simulink library "AF_MDL"  (R2015a)
settings: Solver=ode45  StartTime=0.0  StopTime=10.0  RelTol=1e-3
undefined symbols (not defined in the file or in its folder): AF
libraries: simulink x1
settings Model: Creator=Andrew  LastModifiedBy=Andrew

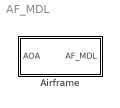
== system AF_MDL ==
  Airframe : Subsystem  mask{AF=AF}
      mask prompts: AF "INPUTS"

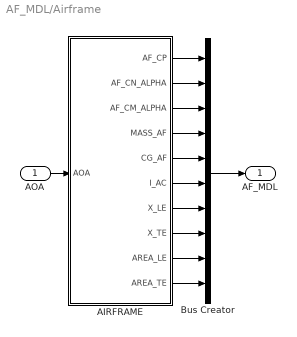
== system AF_MDL/Airframe ==
  AOA : Inport
  AIRFRAME : Subsystem
  Bus Creator : BusCreator  Inputs=10
  AF_MDL : Outport
  wires:
  Bus Creator/1 -> AF_MDL/1
  AIRFRAME/2(AF_CN_ALPHA) -> Bus Creator/2
  AIRFRAME/4(MASS_AF) -> Bus Creator/4
  AIRFRAME/1(AF_CP) -> Bus Creator/1
  AIRFRAME/3(AF_CM_ALPHA) -> Bus Creator/3
  AIRFRAME/5(CG_AF) -> Bus Creator/5
  AIRFRAME/6(I_AC) -> Bus Creator/6
  AOA/1 -> AIRFRAME/1(AOA)
  AIRFRAME/7(X_LE) -> Bus Creator/7
  AIRFRAME/8(X_TE) -> Bus Creator/8
  AIRFRAME/9(AREA_LE) -> Bus Creator/9
  AIRFRAME/10(AREA_TE) -> Bus Creator/10

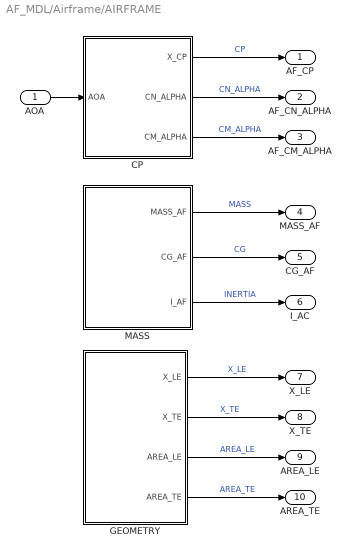
== system AF_MDL/Airframe/AIRFRAME ==
  AOA : Inport
  CP : Subsystem
  GEOMETRY : Subsystem
  MASS : Subsystem
  AF_CP : Outport
  AF_CN_ALPHA : Outport  Port=2
  AF_CM_ALPHA : Outport  Port=3
  MASS_AF : Outport  Port=4
  CG_AF : Outport  Port=5
  I_AC : Outport  Port=6
  X_LE : Outport  Port=7
  X_TE : Outport  Port=8
  AREA_LE : Outport  Port=9
  AREA_TE : Outport  Port=10
  wires:
  CP/1(X_CP) -> AF_CP/1  "CP"
  CP/2(CN_ALPHA) -> AF_CN_ALPHA/1  "CN_ALPHA"
  AOA/1 -> CP/1(AOA)
  CP/3(CM_ALPHA) -> AF_CM_ALPHA/1  "CM_ALPHA"
  MASS/1(MASS_AF) -> MASS_AF/1  "MASS"
  MASS/2(CG_AF) -> CG_AF/1  "CG"
  MASS/3(I_AF) -> I_AC/1  "INERTIA"
  GEOMETRY/1(X_LE) -> X_LE/1  "X_LE"
  GEOMETRY/2(X_TE) -> X_TE/1  "X_TE"
  GEOMETRY/3(AREA_LE) -> AREA_LE/1  "AREA_LE"
  GEOMETRY/4(AREA_TE) -> AREA_TE/1  "AREA_TE"

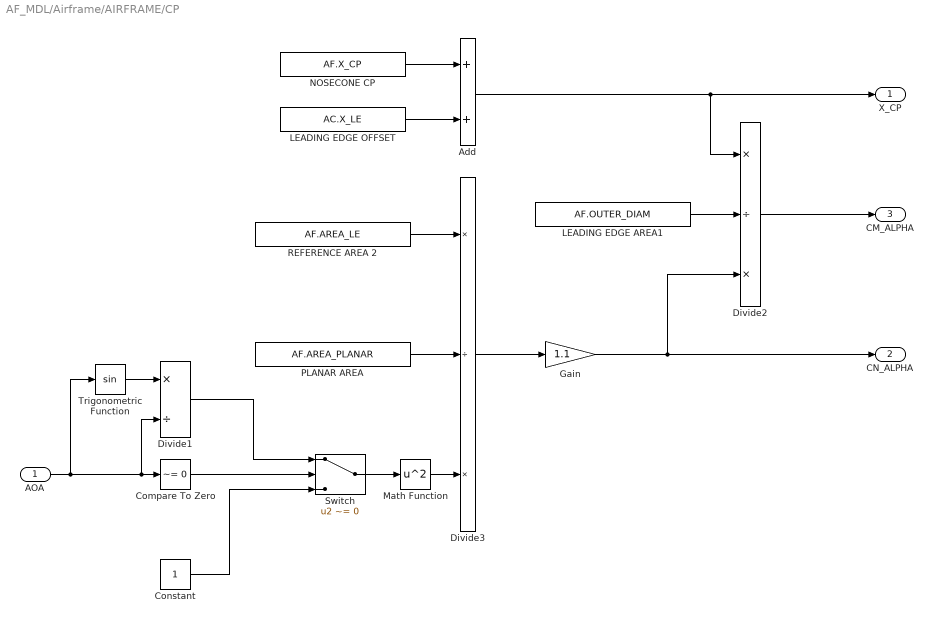
== system AF_MDL/Airframe/AIRFRAME/CP ==
  AOA : Inport
  Add : Sum
  Compare To Zero : simulink/Logic and Bit Operations/Compare To Zero  relop=~=  OutDataTypeStr=boolean
  Constant : Constant
  Divide1 : Product  Inputs=*/
  Divide2 : Product  Inputs=*/*
  Divide3 : Product  Inputs=*/*
  Gain : Gain  Gain=1.1
  LEADING EDGE AREA1 : FromWorkspace  VariableName=AF.OUTER_DIAM
  LEADING EDGE OFFSET : FromWorkspace  VariableName=AC.X_LE
  Math Function : Math  Operator=square  SaturateOnIntegerOverflow=on
  NOSECONE CP : FromWorkspace  VariableName=AF.X_CP
  PLANAR AREA : FromWorkspace  VariableName=AF.AREA_PLANAR
  REFERENCE AREA 2 : FromWorkspace  VariableName=AF.AREA_LE
  Switch : Switch  Criteria=u2 ~= 0
  Trigonometric Function : Trigonometry  OutputSignalType=real
  X_CP : Outport
  CN_ALPHA : Outport  Port=2
  CM_ALPHA : Outport  Port=3
  wires:
  Divide1/1 -> Switch/1
  Trigonometric Function/1 -> Divide1/1
  AOA/1 -> Compare To Zero/1, Divide1/2, Trigonometric Function/1
  Constant/1 -> Switch/3
  Compare To Zero/1 -> Switch/2
  Switch/1 -> Math Function/1
  Add/1 -> Divide2/1, X_CP/1
  LEADING EDGE OFFSET/1 -> Add/2
  NOSECONE CP/1 -> Add/1
  Divide2/1 -> CM_ALPHA/1
  LEADING EDGE AREA1/1 -> Divide2/2
  Math Function/1 -> Divide3/3
  Divide3/1 -> Gain/1
  REFERENCE AREA 2/1 -> Divide3/1
  PLANAR AREA/1 -> Divide3/2
  Gain/1 -> Divide2/3, CN_ALPHA/1

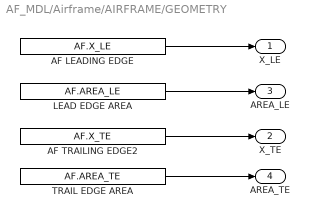
== system AF_MDL/Airframe/AIRFRAME/GEOMETRY ==
  AF LEADING EDGE : Constant  Value=AF.X_LE
  AF TRAILING EDGE2 : Constant  Value=AF.X_TE
  LEAD EDGE AREA : Constant  Value=AF.AREA_LE
  TRAIL EDGE AREA : Constant  Value=AF.AREA_TE
  X_LE : Outport
  X_TE : Outport  Port=2
  AREA_LE : Outport  Port=3
  AREA_TE : Outport  Port=4
  wires:
  TRAIL EDGE AREA/1 -> AREA_TE/1
  AF LEADING EDGE/1 -> X_LE/1
  LEAD EDGE AREA/1 -> AREA_LE/1
  AF TRAILING EDGE2/1 -> X_TE/1

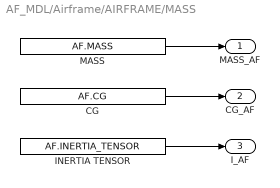
== system AF_MDL/Airframe/AIRFRAME/MASS ==
  CG : Constant  Value=AF.CG
  INERTIA TENSOR : Constant  Value=AF.INERTIA_TENSOR
  MASS : Constant  Value=AF.MASS
  MASS_AF : Outport
  CG_AF : Outport  Port=2
  I_AF : Outport  Port=3
  wires:
  INERTIA TENSOR/1 -> I_AF/1
  MASS/1 -> MASS_AF/1
  CG/1 -> CG_AF/1
